simulink library "Lib_PFSys_GenericThreePhaseMotor_TMATS"  (R2019b)
settings: Solver=ode45  StartTime=0.0  StopTime=10.0  RelTol=1e-3  EnableMultiTasking=on
libraries: $bdroot x1
Description:
  | Thomas Modules
settings Model: Creator=jwchapm2  LastModifiedBy=mebell
settings DataIOCC: LimitDataPoints=on  SaveFormat=Array  ReturnWorkspaceOutputs=off
settings OptimizationCC: ExpressionDepthLimit=2147483647  LifeSpan=inf
settings DebuggingCC: UnderspecifiedInitializationDetection=Classic  MergeDetectMultiDrivingBlocksExec=none  SolverPrmCheckMsg=warning  StateNameClashWarn=warning  SFUnexpectedBacktrackingDiag=warning  SFNoUnconditionalDefaultTransitionDiag=warning  SFExecutionAtInitializationDiag=none  ArithmeticOperatorsInVariantConditions=warning
settings HardwareCC: ProdBitPerPointer=32  ProdBitPerSizeT=32  ProdBitPerPtrDiffT=32  ProdLargestAtomicFloat=None  ProdIntDivRoundTo=Undefined  ProdEndianess=Unspecified  ProdWordSize=32  ProdHWDeviceType=32-bit Generic
settings ModelReferenceCC: PropagateSignalLabelsOutOfModel=off
settings SFSimCC: SimUseLocalCustomCode=off  CustomCodeUndefinedFunction=UseInterfaceOnly
settings RTWCC: RTWUseLocalCustomCode=off
settings CodeAppCC: StateflowObjectComments=on
settings GRTTargetCC: TargetLangStandard=C89/C90 (ANSI)  GeneratePreprocessorConditionals=Disable all
settings ConfigComp: CovMetricSettings=dw  CovHtmlReporting=on  CovSaveCumulativeToWorkspaceVar=on  CovSaveSingleToWorkspaceVar=on  CovExternalEMLEnable=off

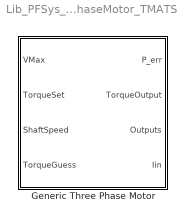
== system Lib_PFSys_GenericThreePhaseMotor_TMATS ==
  Generic Three Phase Motor : Subsystem  mask(Motor){X_C_SpeedVec_M=[0.0 0.1 1.0], Y_C_TorqueVec_M=[0.0 0.1 1.0], T_C_EffArray_M=[0.5 0.5 0.5; 0.5 1.0 1.0; 0.5 1.0 1.0], Ke_M=0.5}
      mask prompts: X_C_SpeedVec_M "X_C_SpeedVec_M - Efficiency Table Speed Vector (X-axis)(nx1)"; Y_C_TorqueVec_M "Y_C_TorqueVec_M - Efficiency Table Torque Vector (Y-axis)(mx1)"; T_C_EffArray_M "T_C_EffArray_M - Efficiency Table Values (Eff = f(i, V)(nxm)"; Ke_M "Ke_M - Motor EMF Constant (V/ rad/s)"
      mask help:
      | This block represents a generic motor with a purely resistive input
      | impedance, and a lumped efficiency/loss model, specified as a lookup table.

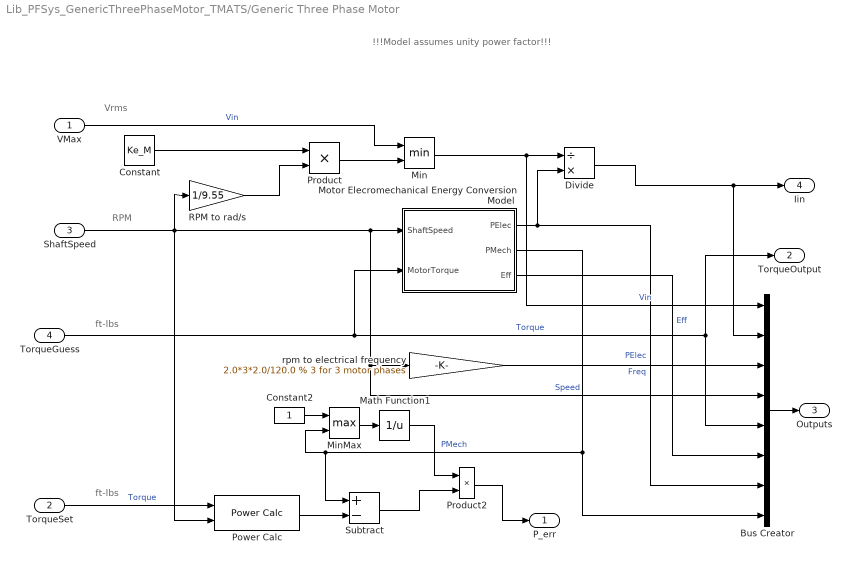
== system Lib_PFSys_GenericThreePhaseMotor_TMATS/Generic Three Phase Motor ==
  note: Vrms
  note: ft-lbs
  note: ft-lbs
  note: RPM
  note: !!!Model assumes unity power factor!!!
  VMax : Inport
  TorqueSet : Inport  Port=2
  ShaftSpeed : Inport  Port=3
  TorqueGuess : Inport  Port=4
  Bus Creator : BusCreator  Inputs=8
  Constant : Constant  Value=Ke_M
  Constant2 : Constant
  Divide : Product  Inputs=/*
  Math Function1 : Math  Operator=reciprocal  SaturateOnIntegerOverflow=on
  Min : MinMax  Inputs=2
  MinMax : MinMax  Function=max  Inputs=2
  Motor Elecromechanical Energy Conversion Model : Subsystem
  Power Calc : $bdroot/Generic Three Phase Motor/Motor Elecromechanical Energy Conversion Model/Power Calc  SystemSampleTime=-1  Latency=0  AutoFrameSizeCalculation=off
  Product : Product
  Product2 : Product
  RPM to rad/s : Gain  Gain=1/9.55
  Subtract : Sum  Inputs=+-
  rpm to electrical frequency : Gain  Gain=2.0*3*2.0/120.0 % 3 for 3 motor phases
  P_err : Outport  VectorParamsAs1DForOutWhenUnconnected=off
  TorqueOutput : Outport  Port=2
  Outputs : Outport  Port=3  VectorParamsAs1DForOutWhenUnconnected=off
  Iin : Outport  Port=4  VectorParamsAs1DForOutWhenUnconnected=off
  wires:
  Motor Elecromechanical Energy Conversion Model/1(PElec) -> Divide/2, Bus Creator/7  "PElec"
  Bus Creator/1 -> Outputs/1
  rpm to electrical frequency/1 -> Bus Creator/3  "Freq"
  TorqueGuess/1 -> Motor Elecromechanical Energy Conversion Model/2(MotorTorque), TorqueOutput/1, Bus Creator/5  "Torque"
  ShaftSpeed/1 -> Motor Elecromechanical Energy Conversion Model/1(ShaftSpeed), Bus Creator/4, rpm to electrical frequency/1, Power Calc/2, RPM to rad/s/1  "Speed"
  Motor Elecromechanical Energy Conversion Model/3(Eff) -> Bus Creator/6  "Eff"
  Motor Elecromechanical Energy Conversion Model/2(PMech) -> Bus Creator/8, Subtract/1, MinMax/2  "PMech"
  Constant/1 -> Product/1
  VMax/1 -> Min/1  "Vin"
  Product/1 -> Min/2
  RPM to rad/s/1 -> Product/2
  Min/1 -> Bus Creator/1, Divide/1  "Vin"
  TorqueSet/1 -> Power Calc/1  "Torque"
  Power Calc/1 -> Subtract/2
  Divide/1 -> Bus Creator/2, Iin/1
  Math Function1/1 -> Product2/1
  Constant2/1 -> MinMax/1
  MinMax/1 -> Math Function1/1
  Product2/1 -> P_err/1
  Subtract/1 -> Product2/2

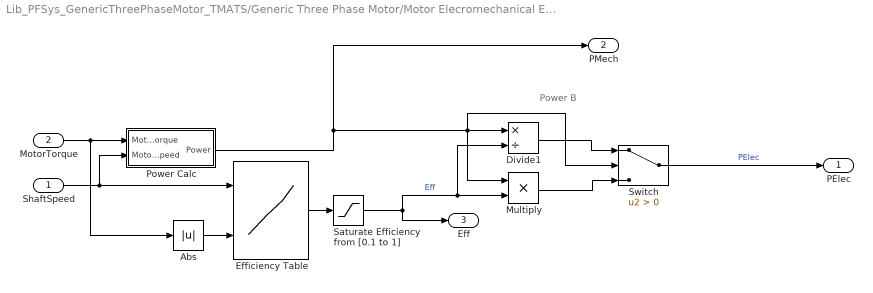
== system Lib_PFSys_GenericThreePhaseMotor_TMATS/Generic Three Phase Motor/Motor Elecromechanical Energy Conversion Model ==
  note: Power B
  ShaftSpeed : Inport
  MotorTorque : Inport  Port=2
  Abs : Abs
  Divide1 : Product  Inputs=*/
  Efficiency Table : Lookup_n-D  BreakpointsForDimension1=X_C_SpeedVec_M  BreakpointsForDimension2=Y_C_TorqueVec_M  Table=T_C_EffArray_M  ExtrapMethod=Clip  InternalRulePriority=Speed  RndMeth=Simplest  InputSameDT=on
  Multiply : Product
  Power Calc : Subsystem
  Saturate Efficiency from [0.1 to 1] : Saturate  UpperLimit=1  LowerLimit=0.1
  Switch : Switch  Criteria=u2 > Threshold
  PElec : Outport  VectorParamsAs1DForOutWhenUnconnected=off
  PMech : Outport  Port=2  VectorParamsAs1DForOutWhenUnconnected=off
  Eff : Outport  Port=3  VectorParamsAs1DForOutWhenUnconnected=off
  wires:
  Efficiency Table/1 -> Saturate Efficiency from [0.1 to 1]/1
  Saturate Efficiency from [0.1 to 1]/1 -> Divide1/2, Multiply/2, Eff/1  "Eff"
  Abs/1 -> Efficiency Table/2
  Switch/1 -> PElec/1  "PElec"
  MotorTorque/1 -> Abs/1, Power Calc/1(MotorTorque)
  ShaftSpeed/1 -> Power Calc/2(MotorSpeed), Efficiency Table/1
  Power Calc/1(Power) -> Switch/2, Multiply/1, Divide1/1, PMech/1
  Divide1/1 -> Switch/1
  Multiply/1 -> Switch/3

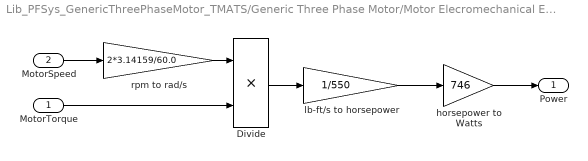
== system Lib_PFSys_GenericThreePhaseMotor_TMATS/Generic Three Phase Motor/Motor Elecromechanical Energy Conversion Model/Power Calc ==
  MotorTorque : Inport
  MotorSpeed : Inport  Port=2
  Divide : Product  Inputs=**
  horsepower to Watts : Gain  Gain=746
  lb-ft/s to horsepower : Gain  Gain=1/550
  rpm to rad/s : Gain  Gain=2*3.14159/60.0
  Power : Outport  VectorParamsAs1DForOutWhenUnconnected=off
  wires:
  MotorSpeed/1 -> rpm to rad/s/1
  Divide/1 -> lb-ft/s to horsepower/1
  lb-ft/s to horsepower/1 -> horsepower to Watts/1
  MotorTorque/1 -> Divide/2
  rpm to rad/s/1 -> Divide/1
  horsepower to Watts/1 -> Power/1
